simulink model "reduced_order_observer_simulation"  (R2016a)
settings: Solver=VariableStepAuto  StartTime=0.0  StopTime=20.0  RelTol=1e-3
values from neighbouring files (symbols this model uses):
  a = obj.a    [System.m]    (also in system_examples.m = [0, -beta*gamma; 1, -(beta+gamma)])
  ap = obj.a*p    [System.m]
  aq = obj.a*q    [System.m]
  b = obj.b    [System.m]    (also in system_examples.m = [alpha ; 1])
  c = obj.c    [System.m]    (also in system_examples.m = [0,1])
  css = eye(size(a))    [System.m]
  dss = [zeros(size(a,1), 1)]    [System.m]
  e_m_lc = e - l*obj.c    [System.m]
  l = place(a22', a12', des_eigs)'    [System.m]
  pt = t(:, 1:psize)    [System.m]
  qt = t(:, psize + 1:end)    [System.m]
  x0 = obj.x0    [System.m]
settings Model: Creator=micah  LastModifiedBy=micah

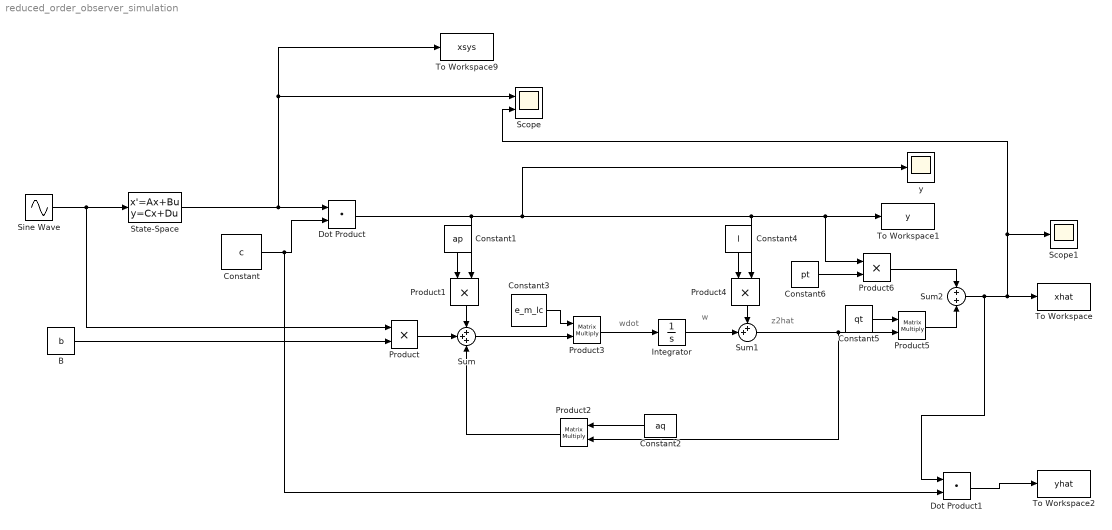
== system reduced_order_observer_simulation ==
  note: z2hat
  note: w
  note: wdot
  B : Constant  Value=b  VectorParams1D=off
  Constant : Constant  Value=c
  Constant1 : Constant  Value=ap
  Constant2 : Constant  Value=aq
  Constant3 : Constant  Value=e_m_lc
  Constant4 : Constant  Value=l
  Constant5 : Constant  Value=qt
  Constant6 : Constant  Value=pt
  Dot Product : DotProduct  InputSameDT=on  OutDataTypeStr=Inherit: Inherit via internal rule
  Dot Product1 : DotProduct  InputSameDT=on  OutDataTypeStr=Inherit: Inherit via internal rule
  Integrator : Integrator
  Product{,1,4,6} (4 alike) : Product
  Product2 : Product  Multiplication=Matrix(*)
  Product3 : Product  Multiplication=Matrix(*)
  Product5 : Product  Multiplication=Matrix(*)
  Scope : Scope  NumInputPorts=2
  Scope1 : Scope
  Sine Wave : Sin  SampleTime=0
  State-Space : StateSpace  A=a  B=b  C=css  D=dss  X0=x0
  Sum : Sum  Inputs=+++
  Sum1 : Sum  Inputs=++|
  Sum2 : Sum  Inputs=+|+
  To Workspace : ToWorkspace  VariableName=xhat  SaveFormat=Structure With Time  SampleTime=-1
  To Workspace1 : ToWorkspace  VariableName=y  SaveFormat=Structure With Time  SampleTime=-1
  To Workspace2 : ToWorkspace  VariableName=yhat  SaveFormat=Structure With Time  SampleTime=-1
  To Workspace9 : ToWorkspace  VariableName=xsys  SaveFormat=Structure With Time  SampleTime=-1
  y : Scope
  wires:
  Sine Wave/1 -> Product/1, State-Space/1
  State-Space/1 -> To Workspace9/1, Scope/1, Dot Product/1
  Constant/1 -> Dot Product1/2, Dot Product/2
  Dot Product/1 -> y/1, To Workspace1/1, Product6/1, Product4/2, Product1/2
  B/1 -> Product/2
  Product/1 -> Sum/2
  Constant1/1 -> Product1/1
  Product1/1 -> Sum/1
  Constant2/1 -> Product2/1
  Product2/1 -> Sum/3
  Sum/1 -> Product3/2
  Constant3/1 -> Product3/1
  Product3/1 -> Integrator/1
  Integrator/1 -> Sum1/2
  Constant4/1 -> Product4/1
  Product4/1 -> Sum1/1
  Sum1/1 -> Product5/2, Product2/2
  Constant5/1 -> Product5/1
  Constant6/1 -> Product6/2
  Product6/1 -> Sum2/1
  Product5/1 -> Sum2/2
  Sum2/1 -> Dot Product1/1, Scope1/1, Scope/2, To Workspace/1
  Dot Product1/1 -> To Workspace2/1
